simulink model "Fuchs_FDFR_simulink_nonlinear"  (R2024a)
settings: Solver=ode4  StartTime=0.0  StopTime=300  FixedStep=0.02  RelTol=1e-3
libraries: vrlib x1
(part 2 of 3)

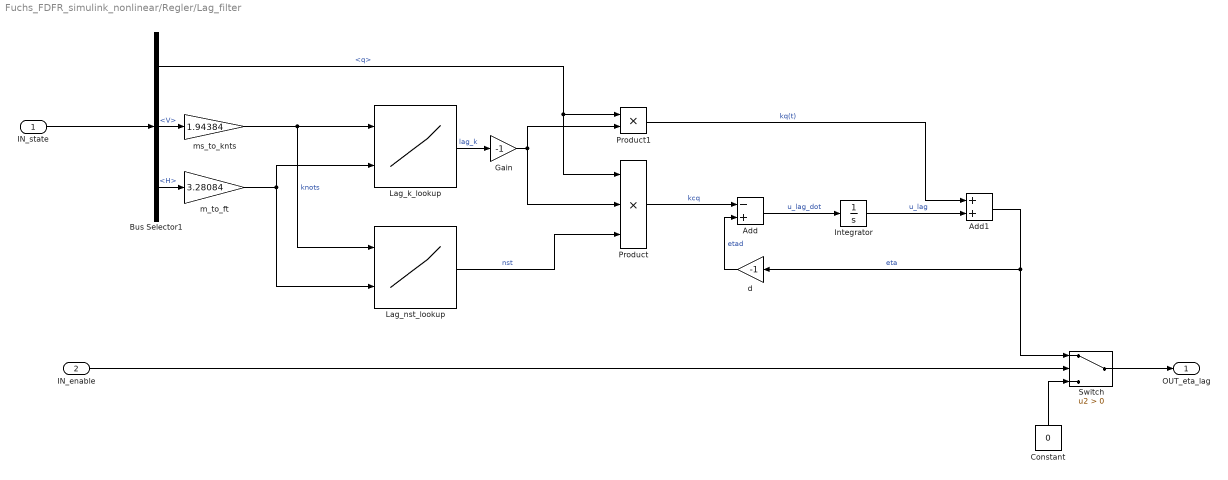
== system Fuchs_FDFR_simulink_nonlinear/Regler/Lag_filter ==
  IN_state : Inport
  IN_enable : Inport  Port=2
  Add : Sum  Inputs=-+
  Add1 : Sum
  Bus Selector1 : BusSelector  OutputSignals=q,V,H
  Constant : Constant  Value=0
  Gain : Gain  Gain=-1
  Integrator : Integrator
  Lag_k_lookup : Lookup_n-D  BreakpointsForDimension1=[300 310 320 330 340 350 360 370 380 390 400 410 420 430 440 450 460 470 480 490 500 510 520 530 540 550 560 570 580 590 600]  BreakpointsForDimension2=[15000 16000 17000 18000 19000 20000 21000 22000 23000 24000 25000 26000 27000 28000 29000 30000 31000 32000 33000 34000 35000 36000 37000 38000 39000 40000 41000 42000 43000 44000 45000]  BreakpointsForDimension3=[5, 7]  Table=[-1.9976095463894787 -2.0753225706470997 -2.1559415937600259 -2.2396262443393251 -2.3265447352480355 -2.416874457996534 -2.5108026232070042 -2.6085269505958921 -2.7102564123159163 -2.8162120339224832 -2.9266277576876485 -3.0417513734830788 -3.1618455229972073 -3.2871887836469087 -3.4180768391974956 -3.5548237448239162 -3.6977632951390516 -3.8472505045914884 -4.0036632106053025 -4.167403810910387 -4.338901147706216 -4.5186125526305929 -4.7070260679838585 -4.904662861308033 -5.1120798522606856 -5.3298725727799674 -5.55867828383793 -5.7991793746562337 -6.0521070731477806 -6.31824549959138 -6.5984360991920656;-1.8616938343219087 -1.9349128093813905 -2.0108325930762532 -2.0896036315492519 -2.1713843790594911 -2.2563418532620276 -2.3446522341515923 -2.4365015098138048 -2.5320861725064434 -2.6316139690000777 -2.7353047095456513 -2.8433911403113479 -2.9561198846473036 -3.07375245910036 -3.1965663707183323 -3.3248563028614129 -3.4589353974850288 -3.5991366426828049 -3.7458143751898691 -3.8993459085568634 -4.0601332988259342 -4.2286052607860043 -4.4052192492712834 -4.5904637215126289 -4.7848605982760191 -4.9889679434493 -5.2033828838939744 -5.42874479379268 -5.665738770429595 -5.9150994313792387 -6.1776150664933622;-1.7381515834523549 -1.8073159743658189 -1.8789935986579911 -1.9533266222840371 -2.0304646969751787 -2.1105654793785957 -2.1937951917988028 -2.2803292273891786 -2.3703528030113623 -2.4640616633737662 -2.5616628404823141 -2.6633754728913814 -2.7694316897356281 -2.8800775650595605 -2.9955741485472753 -3.1161985793967473 -3.2422452907885275 -3.3740273131763576 -3.5118776854863789 -3.6561509842624229 -3.8072249818495894 -3.9655024458796766 -4.1314130936254054 -4.3054157162424316 -4.4880004895379653 -4.6796914897143687 -4.8810494345599507 -5.0926746728252947 -5.3152104470642705 -5.5493464580704845 -5.7958227622448195;-1.6254784670317388 -1.6909760214870373 -1.7588147143269244 -1.8291292244426127 -1.9020612422309693 -1.9777599550822804 -2.0563825727283285 -2.1380948950117991 -2.2230719250001281 -2.3114985307503537 -2.403570159440318 -2.4994936080200638 -2.599487855010048 -2.7037849585853433 -2.8126310266429844 -2.926287265159575 -3.0450311118152036 -3.169157462595797 -3.2989799998979619 -3.4348326315580295 -3.5770710512218131 -3.7260744315755367 -3.882247263186331 -4.046021353067685 -4.2178579986102331 -4.3982503542208757 -4.5877260099174535 -4.7868498032581082 -4.9962268883740864 -5.2165060885570442 -5.4483835618658452;-1.5223894715925512 -1.5845637012290412 -1.648920632427862 -1.7155881561077713 -1.7847007437129427 -1.8563999011015409 -1.9308346608589384 -2.008162115312877 -2.0885479928856756 -2.1721672807950991 -2.2592048975143109 -2.3498564188267204 -2.4443288617678522 -2.5428415312387873 -2.6456269346099157 -2.7529317702156675 -2.8650179962775413 -2.9821639874917278 -3.10466578728725 -3.2328384646104156 -3.3670175850319559 -3.50756080701628 -3.6548496153515724 -3.8092912050294481 -3.9713205303012566 -4.1414025352437074 -4.3200345839615588 -4.5077491105645322 -4.7051165113077387 -4.912748303812382 -5.1313005811233419;-1.4277817029873558 -1.4869380982232081 -1.5481308545308345 -1.6114816924161899 -1.6771185212363175 -1.7451758631507182 -1.8157953143555849 -1.8891260455953531 -1.9653253443022358 -2.0445592010867122 -2.1270029436939359 -2.2128419219562114 -2.3022722477148654 -2.3955015941604976 -2.49275005955443 -2.5942511008518134 -2.700252543355107 -2.8110176731926466 -2.9268264201489211 -3.0479766391799283 -3.1747854998387317 -3.3075909938241748 -3.4467535719626219 -3.5926579231526197 -3.7457149091617365 -3.9063636706818428 -4.075073921744611 -4.252348451496502 -4.4387258544587711 -4.6347835127840771 -4.841140856701907;-1.3407043444842797 -1.3971155654634995 -1.4554275594630151 -1.5157564229805396 -1.5782240856860204 -1.6429587057426336 -1.7100951015545522 -1.7797752216513461 -1.8521486547759856 -1.9273731826142555 -2.0056153779911612 -2.0870512517680644 -2.1718669521072353 -2.2602595202326454 -2.3524377073125358 ...(+15285 chars)]  InternalRulePriority=Speed  RndMeth=Simplest
      settings: InputPortMap=u0,u1
  Lag_nst_lookup : Lookup_n-D  BreakpointsForDimension1=[300 310 320 330 340 350 360 370 380 390 400 410 420 430 440 450 460 470 480 490 500 510 520 530 540 550 560 570 580 590 600]  BreakpointsForDimension2=[15000 16000 17000 18000 19000 20000 21000 22000 23000 24000 25000 26000 27000 28000 29000 30000 31000 32000 33000 34000 35000 36000 37000 38000 39000 40000 41000 42000 43000 44000 45000]  BreakpointsForDimension3=[5, 7]  Table=[-2.4320248547469356 -2.4461261639414227 -2.4596550454821258 -2.4726374662492061 -2.4850979140208085 -2.4970595106053834 -2.5085441131709385 -2.5195724053436019 -2.5301639794038997 -2.5403374107069183 -2.5501103252844062 -2.5594994614464586 -2.5685207260831873 -2.5771892462680395 -2.5855194166815014 -2.5935249433037844 -2.6012188837657151 -2.60861368469661 -2.6157212163649342 -2.6225528048708258 -2.6291192621182158 -2.6354309137671308 -2.6414976253436668 -2.6473288266649222 -2.6529335347188865 -2.6583203751241085 -2.6634976022809056 -2.6684731183143708 -2.6732544908993767 -2.6778489700490349 -2.6822635039402534;-2.3958852472547973 -2.41159254900022 -2.4266496848276637 -2.4410874499950794 -2.4549347489260795 -2.4682187540021014 -2.4809650464465 -2.4931977418044924 -2.5049396021217345 -2.5162121365937051 -2.52703569218478 -2.5374295354890721 -2.5474119269162925 -2.5570001881279936 -2.5662107635175455 -2.5750592764157485 -2.5835605806105342 -2.5917288076896843 -2.5995774106484513 -2.6071192041466462 -2.6143664017510817 -2.6213306504574541 -2.6280230627500969 -2.6344542464271568 -2.6406343323923549 -2.6465730005915344 -2.6522795042522813 -2.6577626925678324 -2.6630310319512454 -2.6680926259728905 -2.672955234082703;-2.3577086166056622 -2.3751412208224592 -2.3918369923067 -2.4078324414866454 -2.4231616674743237 -2.4378565779113242 -2.4519470823692391 -2.4654612631623376 -2.4784255267919066 -2.490864738719476 -2.5028023437368776 -2.5142604738470316 -2.5252600452761227 -2.5358208459942113 -2.5459616149181641 -2.5557001138008371 -2.5650531926678259 -2.5740368495430332 -2.5826662851029476 -2.5909559528136068 -2.5989196050314609 -2.606570335487095 -2.613920618517918 -2.620982345370428 -2.6277668578537736 -2.6342849795927537 -2.6405470450994684 -2.6465629268578672 -2.652342060593607 -2.657893468882929 -2.6632257832376611;-2.3174246624626442 -2.3367108655194886 -2.3551634245327198 -2.3728256280677229 -2.3897376965845609 -2.405937083404174 -2.4214587374007221 -2.436335333223842 -2.4505974738636707 -2.4642738695657909 -2.477391496445704 -2.4899757376131055 -2.5020505091726006 -2.5136383731006693 -2.5247606386946715 -2.5354374540365807 -2.545687888702818 -2.5555300087745265 -2.5649809450537875 -2.5740569552659442 -2.5827734809220426 -2.59114519942555 -2.5991860719310109 -2.6069093873971241 -2.6143278032209607 -2.6214533827922848 -2.6282976302658581 -2.6348715228142185 -2.6411855405929465 -2.6472496946237882 -2.6530735527782894;-2.274955708645471 -2.2962340228664537 -2.3165703140430947 -2.3360159244842236 -2.354618300925015 -2.3724214027149344 -2.3894660554621123 -2.40579025871378 -2.4214294547398509 -2.4364167642663426 -2.4507831940157927 -2.4645578201061311 -2.4777679507002817 -2.490439270757447 -2.5025959712906949 -2.51426086516601 -2.5254554911710767 -2.5362002078262162 -2.5465142781960122 -2.5564159467805339 -2.56592250941403 -2.5750503769713458 -2.5838151335743227 -2.5922315898986348 -2.600313832103569 -2.6080752668403768 -2.6155286627378724 -2.6226861887149155 -2.6295594494272345 -2.6361595181196891 -2.6424969671236829;-2.2302157028569369 -2.2536362736593576 -2.275993207104106 -2.2973474317471694 -2.3177549395108752 -2.3372673349942561 -2.3559323079891037 -2.3737940417153509 -2.3908935670114508 -2.4072690708917031 -2.4229561664146573 -2.437988129619673 -2.4523961083241073 -2.466209306786407 -2.4794551495950827 -2.4921594276125507 -2.5043464283640642 -2.516039052898134 -2.5272589208421881 -2.5380264651241897 -2.5483610176192806 -2.5582808868023785 -2.5678034283375775 -2.5769451094082436 -2.58572156748411 -2.5941476641300292 -2.6022375343831294 -2.6100046321581742 -2.6174617720839159 -2.6246211681238791 -2.6314944692927833;-2.1831090843545424 -2.208835325548697 -2.2333611232094319 -2.2567588354090828 -2.2790945752867509 -2.3004289454752107 -2.3208176654374029 -2.3403121097746076 -2.358959772173 -2.3768046669587721 -2.3938876780784484 -2.4102468635920027 -2.4259177223711097 -2.4409334285635609 -2.4553250384633656 -2.4691216736721935 ...(+15034 chars)]  InternalRulePriority=Speed  RndMeth=Simplest
      settings: InputPortMap=u0,u1
  Product : Product  Inputs=3
  Product1 : Product
  Switch : Switch  Criteria=u2 > Threshold  SaturateOnIntegerOverflow=off  InputSameDT=off
  d : Gain  Gain=-1
  m_to_ft : Gain  Gain=3.28084
  ms_to_knts : Gain  Gain=1.94384
  OUT_eta_lag : Outport
  wires:
  Bus Selector1/2 -> ms_to_knts/1  "<V>"
  Lag_k_lookup/1 -> Gain/1  "lag_k"
  m_to_ft/1 -> Lag_k_lookup/2, Lag_nst_lookup/2
  IN_state/1 -> Bus Selector1/1
  Switch/1 -> OUT_eta_lag/1
  IN_enable/1 -> Switch/2
  Constant/1 -> Switch/3
  Add/1 -> Integrator/1  "u_lag_dot"
  Product/1 -> Add/1  "kcq"
  Integrator/1 -> Add1/2  "u_lag"
  Bus Selector1/1 -> Product/1, Product1/1  "<q>"
  Product1/1 -> Add1/1  "kq(t)"
  Add1/1 -> Switch/1, d/1  "eta"
  d/1 -> Add/2  "etad"
  Lag_nst_lookup/1 -> Product/3  "nst"
  Gain/1 -> Product/2, Product1/2
  ms_to_knts/1 -> Lag_k_lookup/1, Lag_nst_lookup/1  "knots"
  Bus Selector1/3 -> m_to_ft/1  "<H>"

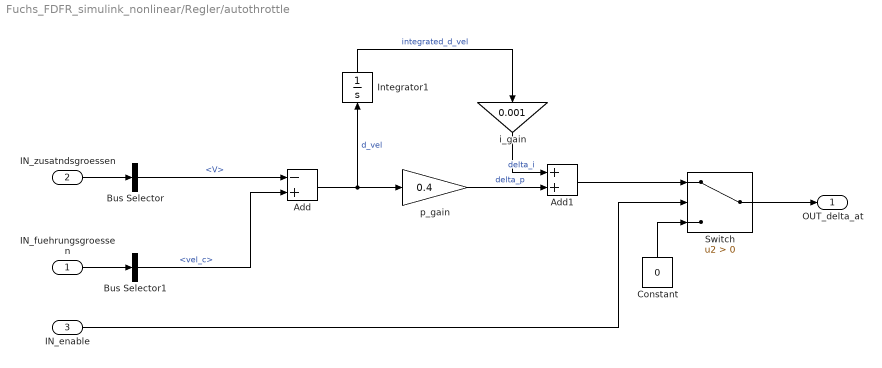
== system Fuchs_FDFR_simulink_nonlinear/Regler/autothrottle ==
  IN_fuehrungsgroessen : Inport
  IN_zusatndsgroessen : Inport  Port=2
  IN_enable : Inport  Port=3
  Add : Sum  Inputs=-+
  Add1 : Sum
  Bus Selector : BusSelector  OutputSignals=V
  Bus Selector1 : BusSelector  OutputSignals=vel_c
  Constant : Constant  Value=0
  Integrator1 : Integrator
  Switch : Switch  Criteria=u2 > Threshold  SaturateOnIntegerOverflow=off  InputSameDT=off
  i_gain : Gain  Gain=0.001
  p_gain : Gain  Gain=0.4
  OUT_delta_at : Outport
  wires:
  IN_zusatndsgroessen/1 -> Bus Selector/1
  Bus Selector/1 -> Add/1  "<V>"
  IN_fuehrungsgroessen/1 -> Bus Selector1/1
  Bus Selector1/1 -> Add/2  "<vel_c>"
  Add/1 -> Integrator1/1, p_gain/1  "d_vel"
  p_gain/1 -> Add1/2  "delta_p"
  Switch/1 -> OUT_delta_at/1
  IN_enable/1 -> Switch/2
  Constant/1 -> Switch/3
  Integrator1/1 -> i_gain/1  "integrated_d_vel"
  i_gain/1 -> Add1/1  "delta_i"
  Add1/1 -> Switch/1

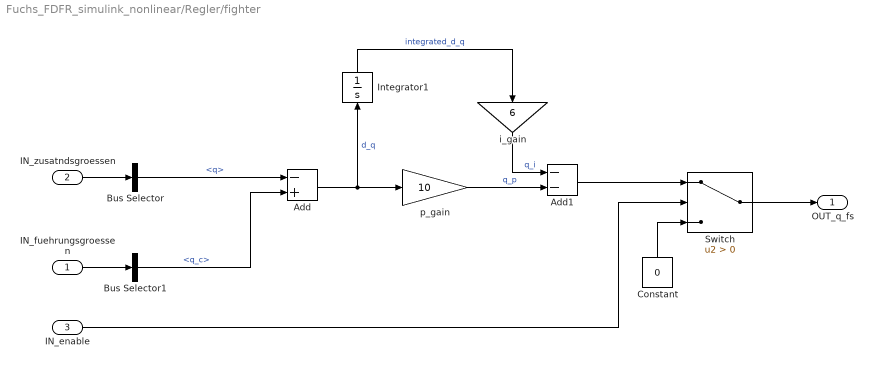
== system Fuchs_FDFR_simulink_nonlinear/Regler/fighter ==
  IN_fuehrungsgroessen : Inport
  IN_zusatndsgroessen : Inport  Port=2
  IN_enable : Inport  Port=3
  Add : Sum  Inputs=-+
  Add1 : Sum  Inputs=--
  Bus Selector : BusSelector  OutputSignals=q
  Bus Selector1 : BusSelector  OutputSignals=q_c
  Constant : Constant  Value=0
  Integrator1 : Integrator
  Switch : Switch  Criteria=u2 > Threshold  SaturateOnIntegerOverflow=off  InputSameDT=off
  i_gain : Gain  Gain=6
  p_gain : Gain  Gain=10
  OUT_q_fs : Outport
  wires:
  IN_zusatndsgroessen/1 -> Bus Selector/1
  Bus Selector/1 -> Add/1  "<q>"
  IN_fuehrungsgroessen/1 -> Bus Selector1/1
  Bus Selector1/1 -> Add/2  "<q_c>"
  Add/1 -> Integrator1/1, p_gain/1  "d_q"
  p_gain/1 -> Add1/2  "q_p"
  Switch/1 -> OUT_q_fs/1
  IN_enable/1 -> Switch/2
  Constant/1 -> Switch/3
  Integrator1/1 -> i_gain/1  "integrated_d_q"
  i_gain/1 -> Add1/1  "q_i"
  Add1/1 -> Switch/1

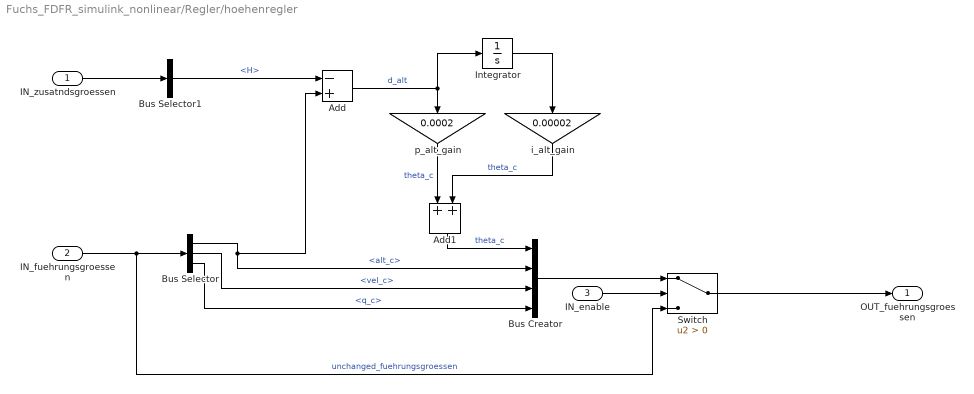
== system Fuchs_FDFR_simulink_nonlinear/Regler/hoehenregler ==
  IN_zusatndsgroessen : Inport
  IN_fuehrungsgroessen : Inport  Port=2
  IN_enable : Inport  Port=3
  Add : Sum  Inputs=-+
  Add1 : Sum
  Bus Creator : BusCreator  Inputs=4
  Bus Selector : BusSelector  OutputSignals=alt_c,vel_c,q_c
  Bus Selector1 : BusSelector  OutputSignals=H
  Integrator : Integrator
  Switch : Switch  Criteria=u2 > Threshold  SaturateOnIntegerOverflow=off  InputSameDT=off
  i_alt_gain : Gain  Gain=0.00002
  p_alt_gain : Gain  Gain=0.0002
  OUT_fuehrungsgroessen : Outport
  wires:
  IN_fuehrungsgroessen/1 -> Switch/3, Bus Selector/1  "unchanged_fuehrungsgroessen"
  Bus Creator/1 -> Switch/1
  IN_enable/1 -> Switch/2
  Switch/1 -> OUT_fuehrungsgroessen/1
  Bus Selector/1 -> Bus Creator/2, Add/2  "<alt_c>"
  IN_zusatndsgroessen/1 -> Bus Selector1/1
  Bus Selector1/1 -> Add/1  "<H>"
  Add/1 -> Integrator/1, p_alt_gain/1  "d_alt"
  Integrator/1 -> i_alt_gain/1
  Add1/1 -> Bus Creator/1  "theta_c"
  p_alt_gain/1 -> Add1/1  "theta_c"
  i_alt_gain/1 -> Add1/2  "theta_c"
  Bus Selector/2 -> Bus Creator/3  "<vel_c>"
  Bus Selector/3 -> Bus Creator/4  "<q_c>"

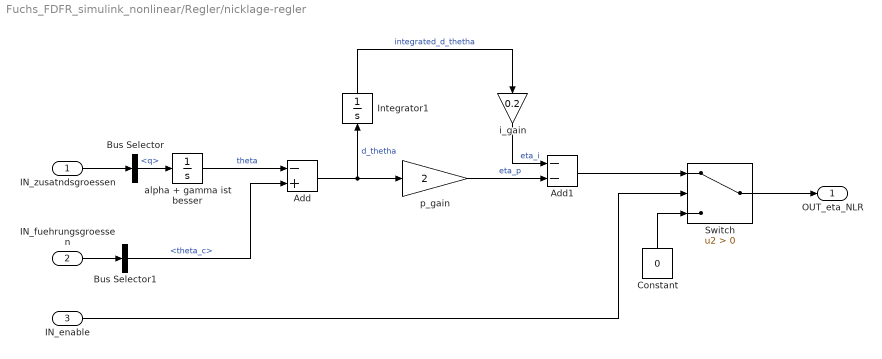
== system Fuchs_FDFR_simulink_nonlinear/Regler/nicklage-regler ==
  IN_zusatndsgroessen : Inport
  IN_fuehrungsgroessen : Inport  Port=2
  IN_enable : Inport  Port=3
  Add : Sum  Inputs=-+
  Add1 : Sum  Inputs=--
  Bus Selector : BusSelector  OutputSignals=q
  Bus Selector1 : BusSelector  OutputSignals=theta_c
  Constant : Constant  Value=0
  Integrator1 : Integrator
  Switch : Switch  Criteria=u2 > Threshold  SaturateOnIntegerOverflow=off  InputSameDT=off
  alpha + gamma ist besser : Integrator
  i_gain : Gain  Gain=0.2
  p_gain : Gain  Gain=2
  OUT_eta_NLR : Outport
  wires:
  IN_zusatndsgroessen/1 -> Bus Selector/1
  Bus Selector/1 -> alpha + gamma ist besser/1  "<q>"
  alpha + gamma ist besser/1 -> Add/1  "theta"
  IN_fuehrungsgroessen/1 -> Bus Selector1/1
  Bus Selector1/1 -> Add/2  "<theta_c>"
  Add/1 -> p_gain/1, Integrator1/1  "d_thetha"
  p_gain/1 -> Add1/2  "eta_p"
  Switch/1 -> OUT_eta_NLR/1
  IN_enable/1 -> Switch/2
  Constant/1 -> Switch/3
  Integrator1/1 -> i_gain/1  "integrated_d_thetha"
  i_gain/1 -> Add1/1  "eta_i"
  Add1/1 -> Switch/1

== system Fuchs_FDFR_simulink_nonlinear/Strecke/Beiwerte ==
  IN_Steuereigaben : Inport
  IN_Zustandsgroessen : Inport  Port=2
  IN_zustandsgroessen_dot : Inport  Port=3
  IN_ac : Inport  Port=4
  Auftriebsbeiwert : Subsystem
  Bus Creator : BusCreator  Inputs=3
  Nickmomentbeiwert : Subsystem
  Widerstandsbeiwert : Subsystem
  OUT_beiwerte : Outport
  wires:
  Bus Creator/1 -> OUT_beiwerte/1  "beiwerte"
  Auftriebsbeiwert/1(OUT_C_A) -> Widerstandsbeiwert/1(IN_C_A), Bus Creator/1  "C_A"
  Widerstandsbeiwert/1(OUT_C_W) -> Bus Creator/2  "C_W"
  Nickmomentbeiwert/1(OUT_C_m) -> Bus Creator/3  "C_m"
  IN_Steuereigaben/1 -> Nickmomentbeiwert/1(IN_steuer), Auftriebsbeiwert/1(IN_steuer)
  IN_Zustandsgroessen/1 -> Nickmomentbeiwert/2(IN_zg), Auftriebsbeiwert/2(IN_zg)
  IN_zustandsgroessen_dot/1 -> Nickmomentbeiwert/4(IN_zustandsgroessen_dot)
  IN_ac/1 -> Nickmomentbeiwert/3(IN_ac), Widerstandsbeiwert/2(IN_ac), Auftriebsbeiwert/3(IN_ac)

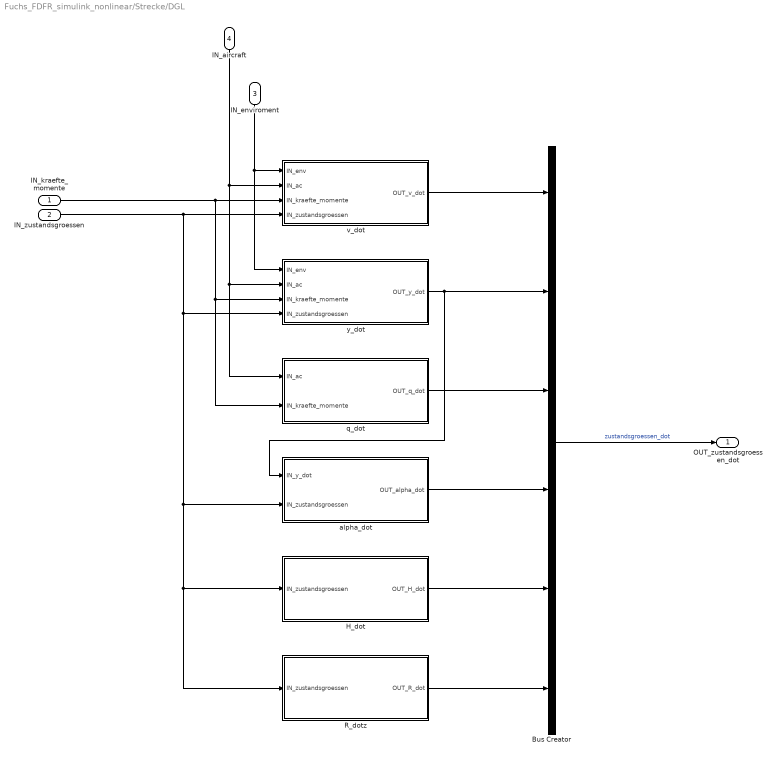
== system Fuchs_FDFR_simulink_nonlinear/Strecke/DGL ==
  IN_kraefte_momente : Inport
  IN_zustandsgroessen : Inport  Port=2
  IN_enviroment : Inport  Port=3
  IN_aircraft : Inport  Port=4
  Bus Creator : BusCreator  Inputs=6
  H_dot : Subsystem
  R_dotz : Subsystem
  alpha_dot : Subsystem
  q_dot : Subsystem
  v_dot : Subsystem
  y_dot : Subsystem
  OUT_zustandsgroessen_dot : Outport
  wires:
  IN_enviroment/1 -> v_dot/1(IN_env), y_dot/1(IN_env)
  IN_aircraft/1 -> y_dot/2(IN_ac), q_dot/1(IN_ac), v_dot/2(IN_ac)
  IN_kraefte_momente/1 -> q_dot/2(IN_kraefte_momente), y_dot/3(IN_kraefte_momente), v_dot/3(IN_kraefte_momente)
  IN_zustandsgroessen/1 -> R_dotz/1(IN_zustandsgroessen), H_dot/1(IN_zustandsgroessen), alpha_dot/2(IN_zustandsgroessen), y_dot/4(IN_zustandsgroessen), v_dot/4(IN_zustandsgroessen)
  y_dot/1(OUT_y_dot) -> alpha_dot/1(IN_y_dot), Bus Creator/2
  v_dot/1(OUT_v_dot) -> Bus Creator/1
  q_dot/1(OUT_q_dot) -> Bus Creator/3
  alpha_dot/1(OUT_alpha_dot) -> Bus Creator/4
  H_dot/1(OUT_H_dot) -> Bus Creator/5
  R_dotz/1(OUT_R_dot) -> Bus Creator/6
  Bus Creator/1 -> OUT_zustandsgroessen_dot/1  "zustandsgroessen_dot"

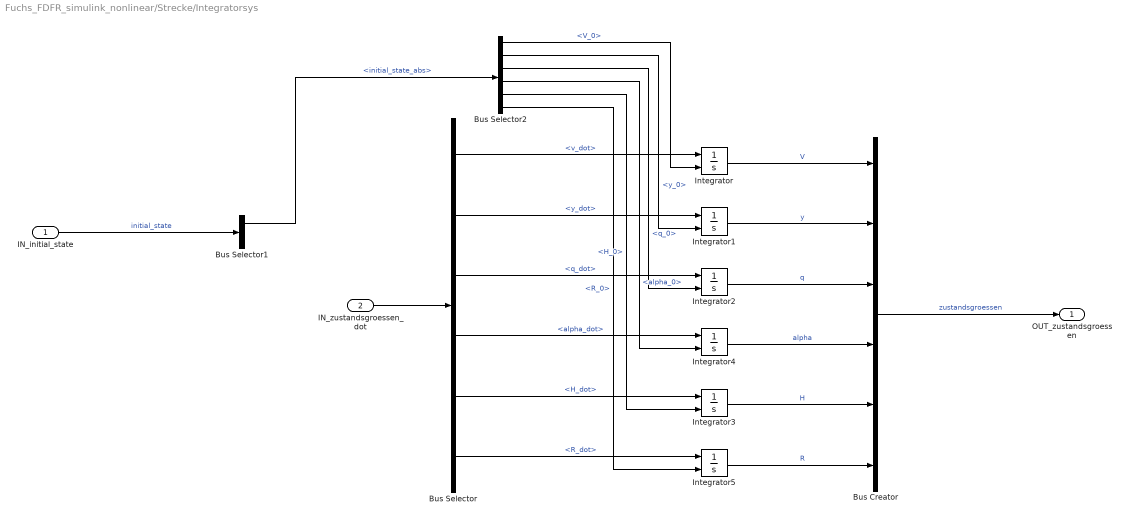
== system Fuchs_FDFR_simulink_nonlinear/Strecke/Integratorsys ==
  IN_initial_state : Inport
  IN_zustandsgroessen_dot : Inport  Port=2
  Bus Creator : BusCreator  Inputs=6
  Bus Selector : BusSelector  OutputSignals=v_dot,y_dot,q_dot,alpha_dot,H_dot,R_dot
  Bus Selector1 : BusSelector  OutputSignals=initial_state_abs,initial_state_dot
  Bus Selector2 : BusSelector  OutputSignals=V_0,y_0,q_0,alpha_0,H_0,R_0
  Integrator{,1..5} (6 alike) : Integrator  InitialConditionSource=external
  OUT_zustandsgroessen : Outport
  wires:
  Bus Creator/1 -> OUT_zustandsgroessen/1  "zustandsgroessen"
  Integrator/1 -> Bus Creator/1  "V"
  Integrator1/1 -> Bus Creator/2  "y"
  Integrator2/1 -> Bus Creator/3  "q"
  Integrator4/1 -> Bus Creator/4  "alpha"
  Integrator3/1 -> Bus Creator/5  "H"
  Integrator5/1 -> Bus Creator/6  "R"
  IN_zustandsgroessen_dot/1 -> Bus Selector/1
  Bus Selector/2 -> Integrator1/1  "<y_dot>"
  Bus Selector/3 -> Integrator2/1  "<q_dot>"
  Bus Selector/4 -> Integrator4/1  "<alpha_dot>"
  Bus Selector/5 -> Integrator3/1  "<H_dot>"
  Bus Selector/6 -> Integrator5/1  "<R_dot>"
  IN_initial_state/1 -> Bus Selector1/1  "initial_state"
  Bus Selector1/1 -> Bus Selector2/1  "<initial_state_abs>"
  Bus Selector2/1 -> Integrator/2  "<V_0>"
  Bus Selector2/3 -> Integrator2/2  "<q_0>"
  Bus Selector2/4 -> Integrator4/2  "<alpha_0>"
  Bus Selector2/5 -> Integrator3/2  "<H_0>"
  Bus Selector2/6 -> Integrator5/2  "<R_0>"
  Bus Selector2/2 -> Integrator1/2  "<y_0>"
  Bus Selector/1 -> Integrator/1  "<v_dot>"

== system Fuchs_FDFR_simulink_nonlinear/Strecke/Kraefte_Momente ==
  IN_steuereingaben : Inport
  IN_beiwerte : Inport  Port=2
  IN_zustandsgroessen : Inport  Port=3
  IN_rho : Inport  Port=4
  IN_ac : Inport  Port=5
  Auftrieb : Subsystem
  Bus Creator : BusCreator  Inputs=4
  Nickmoment : Subsystem
  Schub : Subsystem
  Widerstand : Subsystem
  OUT_kraefte_momente : Outport
  wires:
  Bus Creator/1 -> OUT_kraefte_momente/1  "kraefte_momente"
  Widerstand/1(OUT_W) -> Bus Creator/2  "W"
  Schub/1(OUT_F) -> Bus Creator/4  "F"
  Auftrieb/1(OUT_A) -> Bus Creator/1  "A"
  Nickmoment/1(OUT_M) -> Bus Creator/3  "M"
  IN_beiwerte/1 -> Nickmoment/1(IN_bw), Widerstand/1(IN_bw), Auftrieb/1(IN_bw)  "bw"
  IN_ac/1 -> Schub/2(IN_ac), Nickmoment/3(IN_ac), Widerstand/3(IN_ac), Auftrieb/3(IN_ac)  "ac"
  IN_zustandsgroessen/1 -> Nickmoment/2(IN_zg), Widerstand/2(IN_zg), Auftrieb/2(IN_zg)  "zg"
  IN_rho/1 -> Schub/3(IN_rho), Nickmoment/4(IN_rho), Widerstand/4(IN_rho), Auftrieb/4(IN_rho)  "rho"
  IN_steuereingaben/1 -> Schub/1(IN_steuer)
